simulink model "model_1"  (Simulink 2.20)
settings: Solver=ode45  StartTime=0.0  StopTime=10.0  RelTol=1e-3  AbsTol=1e-6
settings Model: LimitMaxRows=on  ConsistencyChecking=off  RTWPlaceOutputsASAP=off

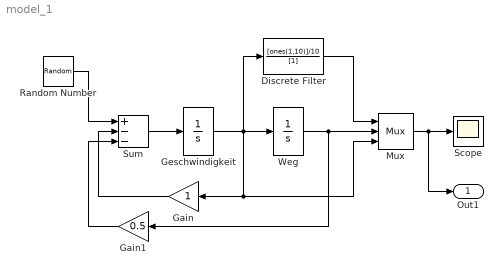
== system model_1 ==
  Discrete Filter : DiscreteFilter  Numerator=[ones(1,10)]/10  Denominator=[1]  SampleTime=0.1
  Gain : Gain  Orientation=left  Gain=1
  Gain1 : Gain  Orientation=left  Gain=0.5
  Geschwindigkeit : Integrator  ExternalReset=none  InitialConditionSource=internal  InitialCondition=0  LimitOutput=off  UpperSaturationLimit=inf  LowerSaturationLimit=-inf  ShowSaturationPort=off  ShowStatePort=off  AbsoluteTolerance=auto
  Mux : Mux  Inputs=3
  Random Number : RandomNumber  Mean=0  Variance=1  Seed=0  SampleTime=-1
  Scope : Scope
      settings: TickLabels=on  TimeRange=auto  YMin=-5  YMax=5  SaveToWorkspace=off  SaveName=ScopeData
  Sum : Sum  Inputs=+--
  Weg : Integrator  ExternalReset=none  InitialConditionSource=internal  InitialCondition=0  LimitOutput=off  UpperSaturationLimit=inf  LowerSaturationLimit=-inf  ShowSaturationPort=off  ShowStatePort=off  AbsoluteTolerance=auto
  Out1 : Outport  Port=1
  wires:
  Random Number/1 -> Sum/1
  Sum/1 -> Geschwindigkeit/1
  Gain/1 -> Sum/2
  Geschwindigkeit/1 -> Weg/1, Discrete Filter/1, Gain/1, Mux/3
  Gain1/1 -> Sum/3
  Weg/1 -> Gain1/1, Mux/2
  Discrete Filter/1 -> Mux/1
  Mux/1 -> Scope/1, Out1/1
